simulink model "simulink_nodes"  (R2021a)
settings: Solver=VariableStepAuto  StartTime=0.0  StopTime=Episode_time  FixedStep=1e-4  MaxStep=TS  RelTol=1e-4
model workspace (MAT data in the model file):
  SL_ROS_VariableLengthArrays_MaxSizes.CommonInfo.ArrayTruncateAction = 'EmitWarning'
  SL_ROS_VariableLengthArrays_MaxSizes.MsgTypeMap = containers.Map
  SL_ROS_VariableLengthArrays_MaxSizes.MsgTypeMap.serialization.keys = {'std_msgs/Float32MultiArray', 'std_msgs/MultiArrayDimension'}
  SL_ROS_VariableLengthArrays_MaxSizes.MsgTypeMap.serialization.values{1}.PropertyName = 'Data'
  SL_ROS_VariableLengthArrays_MaxSizes.MsgTypeMap.serialization.values{1}.DataType = 'single'
  SL_ROS_VariableLengthArrays_MaxSizes.MsgTypeMap.serialization.values{1}.MaxLength = 4
  SL_ROS_VariableLengthArrays_MaxSizes.MsgTypeMap.serialization.values{2}.PropertyName = 'Label'
  SL_ROS_VariableLengthArrays_MaxSizes.MsgTypeMap.serialization.values{2}.DataType = 'uint8'
  SL_ROS_VariableLengthArrays_MaxSizes.MsgTypeMap.serialization.values{2}.MaxLength = 4
  SL_ROS_VariableLengthArrays_MaxSizes.MsgTypeMap.serialization.uniformity = 0
  SL_ROS_VariableLengthArrays_MaxSizes.MsgTypeMap.serialization.keyType = 'char'
  SL_ROS_VariableLengthArrays_MaxSizes.MsgTypeMap.serialization.valueType = 'any'
values from neighbouring files (symbols this model uses):
  Episode_time = 4    [matlab_node.m]
undefined symbols (not defined in the file or in its folder): Data, Data_SL_Info, X, Y, Z
libraries: sm_lib x10, robotlib x7, nesl_utility x6, simulink x1
settings Model: Creator=giulio  LastModifiedBy=giulio
settings SolverCC: NumberNewtonIterations=4  SolverResetMethod=Robust
settings OptimizationCC: EnhancedBackFolding=on  PassReuseOutputArgsAs=Individual arguments  ZeroExternalMemoryAtStartup=off  ZeroInternalMemoryAtStartup=off  MaxStackSize=64  OptimizeBlockOrder=speed  DifferentSizesBufferReuse=on  OptimizationCustomize=off  EfficientTunableParamExpr=on
settings DebuggingCC: ParameterTunabilityLossMsg=error
settings HardwareCC: ProdBitPerPointer=32  ProdBitPerSizeT=32  ProdBitPerPtrDiffT=32  ProdLargestAtomicFloat=None  ProdIntDivRoundTo=Undefined  ProdEndianess=Unspecified  ProdWordSize=32  ProdHWDeviceType=Generic->Unspecified (assume 32-bit Generic)  UseEmbeddedCoderFeatures=off
settings SFSimCC: MATLABDynamicMemAlloc=off
settings RTWCC: SystemTargetFile=ert.tlc  HardwareBoard=Robot Operating System (ROS)  TLCOptions="-aInlineSetEventsForThisBaseRateFcn=TLC_FALSE -aSuppressMultiTaskScheduler=TLC_FALSE  -aRateBasedStepFcn=0"  TemplateMakefile=ert_default_tmf  Toolchain=Catkin  TargetLang=C++
settings CodeAppCC: ForceParamTrailComments=on  IgnoreCustomStorageClasses=off  OperatorAnnotations=on  SimulinkDataObjDesc=on  SFDataObjDesc=on  InsertBlockDesc=on
settings ERTTargetCC: SupportNonInlinedSFcns=on  ERTCustomFileTemplate=rostime_codertarget_file_process.tlc

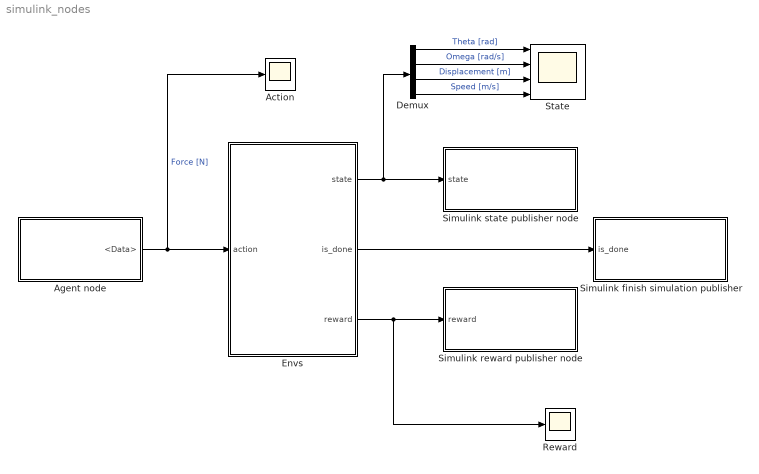
== system simulink_nodes ==
  Action : Scope
  Agent node : Subsystem
  Demux : Demux
  Envs : Subsystem
  Reward : Scope
  Simulink finish simulation publisher : Subsystem
  Simulink reward publisher node : Subsystem
  Simulink state publisher node : Subsystem
  State : Scope  NumInputPorts=4
  wires:
  Envs/1(state) -> Demux/1, Simulink state publisher node/1(state)
  Envs/2(is_done) -> Simulink finish simulation publisher/1(is_done)
  Envs/3(reward) -> Reward/1, Simulink reward publisher node/1(reward)
  Agent node/1(<Data>) -> Action/1, Envs/1(action)  "Force [N]"
  Demux/1 -> State/1  "Theta [rad]"
  Demux/2 -> State/2  "Omega [rad/s]"
  Demux/3 -> State/3  "Displacement [m]"
  Demux/4 -> State/4  "Speed [m/s]"

== system simulink_nodes/Agent node ==
  Bus Selector : BusSelector  OutputSignals=Data
  Subscribe : robotlib/Subscribe  topicSource=Specify your own  topic=/agent_action  messageType=std_msgs/Float32  SampleTime=-1  legacyBusStruct=off  messageQueueLength=1
  Terminator : Terminator
  <Data> : Outport
  wires:
  Bus Selector/1 -> <Data>/1  "<Data>"
  Subscribe/1 -> Terminator/1
  Subscribe/2 -> Bus Selector/1

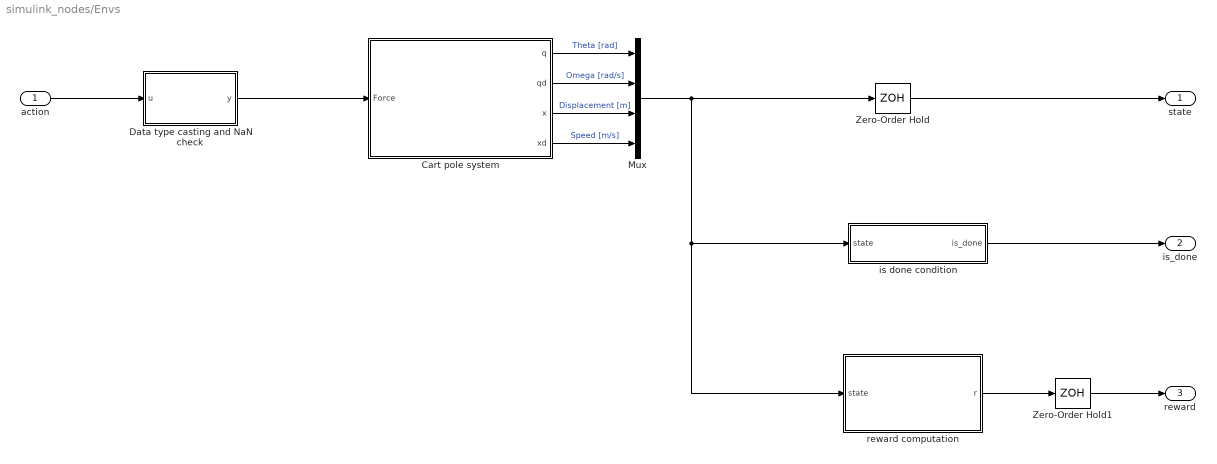
== system simulink_nodes/Envs ==
  action : Inport
  Cart pole system : Subsystem  mask(Cart pole system){mp=0.5, mc=3, bound=15, x_limit=0.5}
      mask prompts: mp "Pole mass [kg]"; mc "Cart pole [kg]"; bound "Pole boundaries [deg]"; x_limit "Cart boundaries [m]"
      mask help: Invertend pendulum on moving base.
      mask DialogControl ParameterGroupVar Prompt: System parameters
      mask Display: image('$imagefile'); % Use "Edit Image" on toolstrip to change.
  Data type casting and NaN check : Subsystem
  Mux : Mux
  Zero-Order Hold : ZeroOrderHold  SampleTime=-1
  Zero-Order Hold1 : ZeroOrderHold  SampleTime=-1
  is done condition : Subsystem  mask{T_sim=Episode_time, x_limit=0.5}
      mask prompts: T_sim "SImulation lenght [s]"; x_limit "X limit [m]"
  reward computation : Subsystem  mask{k_xdisp=100, k_error=20, x_limit=0.5, k_good_angle=10}
      mask prompts: k_xdisp "Displacement penality gain [-]"; k_error "Error angle penalty [-]"; x_limit "x limit [m]"; k_good_angle "Positive gain for good angle [-]"
  state : Outport
  is_done : Outport  Port=2
  reward : Outport  Port=3
  wires:
  Cart pole system/1(q) -> Mux/1  "Theta [rad]"
  Cart pole system/2(qd) -> Mux/2  "Omega [rad/s]"
  Cart pole system/3(x) -> Mux/3  "Displacement [m]"
  Cart pole system/4(xd) -> Mux/4  "Speed [m/s]"
  is done condition/1(is_done) -> is_done/1
  reward computation/1(r) -> Zero-Order Hold1/1
  Mux/1 -> reward computation/1(state), is done condition/1(state), Zero-Order Hold/1
  action/1 -> Data type casting and NaN check/1(u)
  Data type casting and NaN check/1(y) -> Cart pole system/1(Force)
  Zero-Order Hold/1 -> state/1
  Zero-Order Hold1/1 -> reward/1

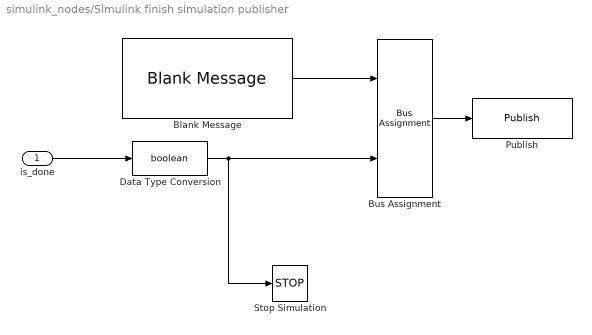
== system simulink_nodes/Simulink finish simulation publisher ==
  is_done : Inport
  Blank Message : robotlib/Blank Message  messageClass=Message  entityType=std_msgs/Bool  messageType=std_msgs/Bool  SampleTime=inf  legacyBusStruct=off
  Bus Assignment : BusAssignment  AssignedSignals=Data
  Data Type Conversion : DataTypeConversion  OutDataTypeStr=boolean
  Publish : robotlib/Publish  topicSource=Specify your own  topic=/is_done  messageType=std_msgs/Bool  legacyBusStruct=off  messageQueueLength=1
  Stop Simulation : Stop
  wires:
  Bus Assignment/1 -> Publish/1
  Blank Message/1 -> Bus Assignment/1
  is_done/1 -> Data Type Conversion/1
  Data Type Conversion/1 -> Stop Simulation/1, Bus Assignment/2

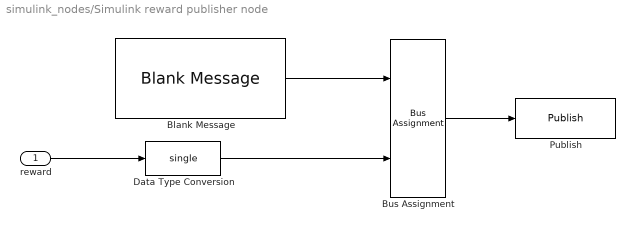
== system simulink_nodes/Simulink reward publisher node ==
  reward : Inport
  Blank Message : robotlib/Blank Message  messageClass=Message  entityType=std_msgs/Float32  messageType=std_msgs/Float32  SampleTime=inf  legacyBusStruct=off
  Bus Assignment : BusAssignment  AssignedSignals=Data
  Data Type Conversion : DataTypeConversion  OutDataTypeStr=single
  Publish : robotlib/Publish  topicSource=Specify your own  topic=/reward  messageType=std_msgs/Float32  legacyBusStruct=off  messageQueueLength=1
  wires:
  Data Type Conversion/1 -> Bus Assignment/2
  Blank Message/1 -> Bus Assignment/1
  Bus Assignment/1 -> Publish/1
  reward/1 -> Data Type Conversion/1

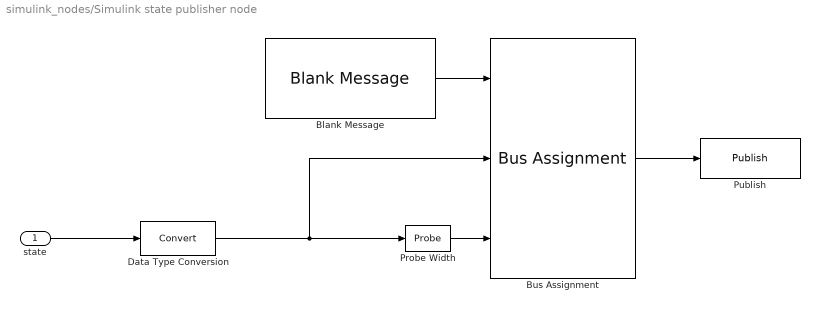
== system simulink_nodes/Simulink state publisher node ==
  state : Inport
  Blank Message : robotlib/Blank Message  messageClass=Message  entityType=std_msgs/Float32MultiArray  messageType=std_msgs/Float32MultiArray  SampleTime=inf  legacyBusStruct=off
  Bus Assignment : BusAssignment  AssignedSignals=Data,Data_SL_Info.CurrentLength
  Data Type Conversion : DataTypeConversion
  Probe Width : Probe  ProbeSampleTime=off  ProbeComplexSignal=off  ProbeWidthDataType=uint32
  Publish : robotlib/Publish  topicSource=Specify your own  topic=/state  messageType=std_msgs/Float32MultiArray  legacyBusStruct=off  messageQueueLength=1
  wires:
  Bus Assignment/1 -> Publish/1
  Probe Width/1 -> Bus Assignment/3
  Blank Message/1 -> Bus Assignment/1
  Data Type Conversion/1 -> Bus Assignment/2, Probe Width/1
  state/1 -> Data Type Conversion/1

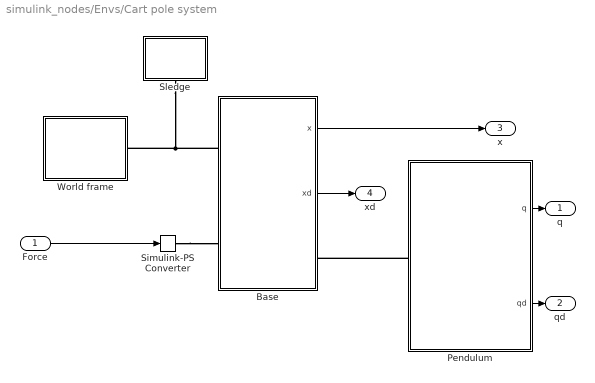
== system simulink_nodes/Envs/Cart pole system ==
  Force : Inport
  Base : Subsystem
  Pendulum : Subsystem
  Simulink-PS Converter : nesl_utility/Simulink-PS Converter  PhysicalDomain=network_engine_domain  SubClassName=ps_input  LeftPortType=input  RightPortType=output  PseudoPeriodic=off  Frequencies=[]  NoiseDistribution=none  NoiseParameters=[]  Unit=1  AffineConversion=off  FilteringAndDerivatives=filter  SimscapeFilterOrder=2  InputFilterTimeConstant=0.001  UdotUserProvided=0
      settings: SourceProductBaseCode=PW,SS
  Sledge : Subsystem
  World frame : Subsystem
  q : Outport
  qd : Outport  Port=2
  x : Outport  Port=3
  xd : Outport  Port=4
  wires:
  Pendulum/1(q) -> q/1
  Pendulum/2(qd) -> qd/1
  Base/2(xd) -> xd/1
  Force/1 -> Simulink-PS Converter/1
  Base/1(x) -> x/1
  connections:
  Simulink-PS Converter/RConn1 -- Base/LConn2
  Pendulum/LConn1 -- Base/RConn1
  Base/LConn1 -- World frame/RConn1 -- Sledge/LConn1

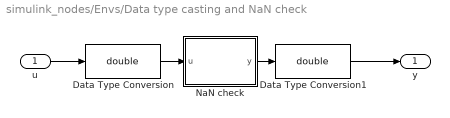
== system simulink_nodes/Envs/Data type casting and NaN check ==
  u : Inport
  Data Type Conversion : DataTypeConversion  OutDataTypeStr=double
  Data Type Conversion1 : DataTypeConversion  OutDataTypeStr=double
  NaN check : MATLAB Function  TreatAsAtomicUnit=on
  y : Outport
  wires:
  NaN check/1(y) -> Data Type Conversion1/1
  Data Type Conversion/1 -> NaN check/1(u)
  u/1 -> Data Type Conversion/1
  Data Type Conversion1/1 -> y/1

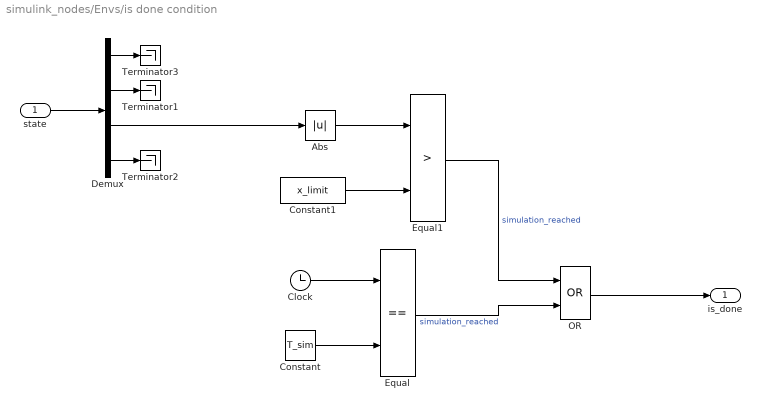
== system simulink_nodes/Envs/is done condition ==
  state : Inport
  Abs : Abs
  Clock : Clock
  Constant : Constant  Value=T_sim
  Constant1 : Constant  Value=x_limit
  Demux : Demux
  Equal : RelationalOperator  Operator===  OutDataTypeStr=boolean  RndMeth=Simplest
  Equal1 : RelationalOperator  Operator=>  OutDataTypeStr=boolean  RndMeth=Simplest
  OR : Logic  Operator=OR  AllPortsSameDT=off  OutDataTypeStr=boolean
  Terminator1 : Terminator
  Terminator2 : Terminator
  Terminator3 : Terminator
  is_done : Outport
  wires:
  Constant/1 -> Equal/2
  Clock/1 -> Equal/1
  state/1 -> Demux/1
  Equal/1 -> OR/2  "simulation_reached"
  OR/1 -> is_done/1
  Demux/3 -> Abs/1
  Abs/1 -> Equal1/1
  Constant1/1 -> Equal1/2
  Equal1/1 -> OR/1  "simulation_reached"
  Demux/2 -> Terminator1/1
  Demux/4 -> Terminator2/1
  Demux/1 -> Terminator3/1

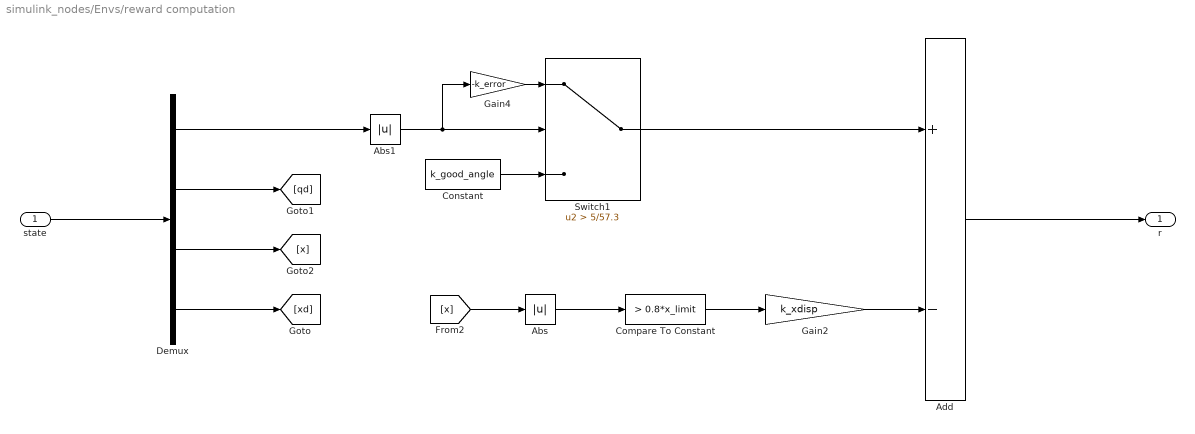
== system simulink_nodes/Envs/reward computation ==
  state : Inport
  Abs : Abs
  Abs1 : Abs
  Add : Sum  Inputs=+-
  Compare To Constant : simulink/Logic and Bit Operations/Compare To Constant  relop=>  const=0.8*x_limit  OutDataTypeStr=boolean
  Constant : Constant  Value=k_good_angle
  Demux : Demux
  Gain2 : Gain  Gain=k_xdisp
  Gain4 : Gain  Gain=-k_error
  Switch1 : Switch  Criteria=u2 > Threshold  Threshold=5/57.3
  r : Outport
  wires:
  state/1 -> Demux/1
  Abs/1 -> Compare To Constant/1
  Add/1 -> r/1
  Switch1/1 -> Add/1
  Demux/1 -> Abs1/1
  Demux/4 -> [xd]
  Demux/3 -> [x]
  Constant/1 -> Switch1/3
  Compare To Constant/1 -> Gain2/1
  Demux/2 -> [qd]
  [x] -> Abs/1
  Gain2/1 -> Add/2
  Abs1/1 -> Gain4/1, Switch1/2
  Gain4/1 -> Switch1/1

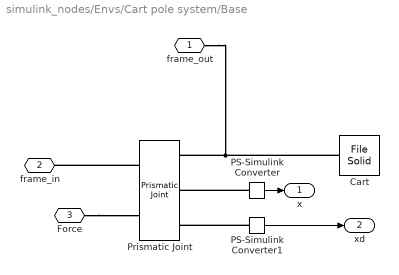
== system simulink_nodes/Envs/Cart pole system/Base ==
  Cart : sm_lib/Body Elements/File Solid  ExtGeomFileName=/home/giulio/rl_prj/simulink/BASE.STEP  UnitType=FromFile  ExtGeomFileUnits=m  StepReaderType=HEX  ExportConvexHullGeometry=off  InertiaType=PointMass  Mass=mc  MassUnits=kg  CenterOfMass=[0 0 0]  CenterOfMassUnits=m  MomentsOfInertia=[1 1 1]  MomentsOfInertiaUnits=kg*m^2  ProductsOfInertia=[0 0 0]  ProductsOfInertiaUnits=kg*m^2  BasedOnType=DensityFromFile  Density=1000  DensityUnits=kg/m^3  DoExposeReferenceFrame=on  SerializedFrames=<Frames/>  GraphicType=FromGeometry  MarkerShape=Sphere  MarkerSize=10  GraphicVisPropType=SimpleVisualProperties  GraphicDiffuseColor=[0.8 0.0 0.2]  GraphicSpecularColor=[0.5 0.5 0.5 1.0]  GraphicAmbientColor=[0.15 0.15 0.15 1.0]  GraphicEmissiveColor=[0.0 0.0 0.0 1.0]  GraphicShininess=75  GraphicOpacity=1.0
  PS-Simulink Converter : nesl_utility/PS-Simulink Converter  PhysicalDomain=network_engine_domain  SubClassName=ps_output  LeftPortType=input  RightPortType=output  PseudoPeriodic=off  Frequencies=[]  Unit=inherit  AffineConversion=off
      settings: SourceProductBaseCode=PW,SS
  PS-Simulink Converter1 : nesl_utility/PS-Simulink Converter  PhysicalDomain=network_engine_domain  SubClassName=ps_output  LeftPortType=input  RightPortType=output  PseudoPeriodic=off  Frequencies=[]  Unit=inherit  AffineConversion=off
      settings: SourceProductBaseCode=PW,SS
  Prismatic Joint : sm_lib/Joints/Prismatic Joint  JointMode=Normal  SenseConstraintForce=off  SenseConstraintForceX=off  SenseConstraintForceY=off  SenseConstraintForceZ=off  SenseConstraintTorque=off  SenseConstraintTorqueX=off  SenseConstraintTorqueY=off  SenseConstraintTorqueZ=off  SenseTotalForce=off  SenseTotalForceX=off  SenseTotalForceY=off  SenseTotalForceZ=off  SenseTotalTorque=off  SenseTotalTorqueX=off  SenseTotalTorqueY=off  SenseTotalTorqueZ=off  CompositeWrenchDir=FollowerOnBase  CompositeWrenchFrame=BaseFrame  EquilibriumPosition=0  EquilibriumPositionUnits=m  SpringStiffness=0  SpringStiffnessUnits=N/m  DampingCoefficient=0  DampingCoefficientUnits=N/(m/s)  TorqueActuationMode=InputTorque  MotionActuationMode=ComputedMotion  SensePosition=on  SenseVelocity=on  SenseAcceleration=off  SenseTorqueForce=off  SenseLowerLimitTorqueForce=off  SenseUpperLimitTorqueForce=off  LowerLimitSpecify=off  LowerLimitBound=-1  LowerLimitBoundUnits=m  LowerLimitStiffness=1e6  LowerLimitStiffnessUnits=N/m  LowerLimitDamping=1e3  LowerLimitDampingUnits=N/(m/s)  LowerLimitTransitionRegionWidth=1e-4  LowerLimitTransitionRegionWidthUnits=m  UpperLimitSpecify=off  UpperLimitBound=1  UpperLimitBoundUnits=m  UpperLimitStiffness=1e6  UpperLimitStiffnessUnits=N/m  UpperLimitDamping=1e3  UpperLimitDampingUnits=N/(m/s)  UpperLimitTransitionRegionWidth=1e-4  UpperLimitTransitionRegionWidthUnits=m  PositionTargetSpecify=on  PositionTargetPriority=Low  PositionTargetValue=0.4*x_limit*randn(1)  PositionTargetValueUnits=m  VelocityTargetSpecify=off  VelocityTargetPriority=Low  VelocityTargetValue=randn(1)  VelocityTargetValueUnits=m/s
  frame_out : PMIOPort  Side=Right
  frame_in : PMIOPort  Port=2  Side=Left
  Force : PMIOPort  Port=3  Side=Left
  x : Outport
  xd : Outport  Port=2
  wires:
  PS-Simulink Converter/1 -> x/1
  PS-Simulink Converter1/1 -> xd/1
  connections:
  Prismatic Joint/LConn1 -- frame_in/RConn1
  Force/RConn1 -- Prismatic Joint/LConn2
  frame_out/RConn1 -- Cart/RConn1 -- Prismatic Joint/RConn1
  PS-Simulink Converter/LConn1 -- Prismatic Joint/RConn2
  PS-Simulink Converter1/LConn1 -- Prismatic Joint/RConn3

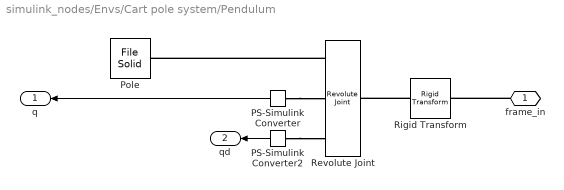
== system simulink_nodes/Envs/Cart pole system/Pendulum ==
  PS-Simulink Converter : nesl_utility/PS-Simulink Converter  PhysicalDomain=network_engine_domain  SubClassName=ps_output  LeftPortType=input  RightPortType=output  PseudoPeriodic=off  Frequencies=[]  Unit=inherit  AffineConversion=off
      settings: SourceProductBaseCode=PW,SS
  PS-Simulink Converter2 : nesl_utility/PS-Simulink Converter  PhysicalDomain=network_engine_domain  SubClassName=ps_output  LeftPortType=input  RightPortType=output  PseudoPeriodic=off  Frequencies=[]  Unit=inherit  AffineConversion=off
      settings: SourceProductBaseCode=PW,SS
  Pole : sm_lib/Body Elements/File Solid  ExtGeomFileName=/home/giulio/rl_prj/simulink/PEND.STEP  UnitType=FromFile  ExtGeomFileUnits=m  StepReaderType=HEX  ExportConvexHullGeometry=off  InertiaType=CalculateFromGeometry  Mass=mp  MassUnits=kg  CenterOfMass=[0 0 0]  CenterOfMassUnits=m  MomentsOfInertia=[1 1 1]  MomentsOfInertiaUnits=kg*m^2  ProductsOfInertia=[0 0 0]  ProductsOfInertiaUnits=kg*m^2  BasedOnType=Mass  Density=1000  DensityUnits=kg/m^3  DoExposeReferenceFrame=on  SerializedFrames=<Frames/>  GraphicType=FromGeometry  MarkerShape=Sphere  MarkerSize=10  GraphicVisPropType=SimpleVisualProperties  GraphicDiffuseColor=[0.0 0.2 0.6]  GraphicSpecularColor=[0.5 0.5 0.5 1.0]  GraphicAmbientColor=[0.15 0.15 0.15 1.0]  GraphicEmissiveColor=[0.0 0.0 0.0 1.0]  GraphicShininess=75  GraphicOpacity=1.0
  Revolute Joint : sm_lib/Joints/Revolute Joint  JointMode=Normal  SenseConstraintForce=off  SenseConstraintForceX=off  SenseConstraintForceY=off  SenseConstraintForceZ=off  SenseConstraintTorque=off  SenseConstraintTorqueX=off  SenseConstraintTorqueY=off  SenseConstraintTorqueZ=off  SenseTotalForce=off  SenseTotalForceX=off  SenseTotalForceY=off  SenseTotalForceZ=off  SenseTotalTorque=off  SenseTotalTorqueX=off  SenseTotalTorqueY=off  SenseTotalTorqueZ=off  CompositeWrenchDir=FollowerOnBase  CompositeWrenchFrame=BaseFrame  EquilibriumPosition=0  EquilibriumPositionUnits=deg  SpringStiffness=0  SpringStiffnessUnits=N*m/deg  DampingCoefficient=0  DampingCoefficientUnits=N*m/(deg/s)  TorqueActuationMode=NoTorque  MotionActuationMode=ComputedMotion  SensePosition=on  SenseVelocity=on  SenseAcceleration=off  SenseTorqueForce=off  SenseLowerLimitTorqueForce=off  SenseUpperLimitTorqueForce=off  LowerLimitSpecify=on  LowerLimitBound=-bound  LowerLimitBoundUnits=deg  LowerLimitStiffness=1e4  LowerLimitStiffnessUnits=N*m/deg  LowerLimitDamping=10  LowerLimitDampingUnits=N*m/(deg/s)  LowerLimitTransitionRegionWidth=0.1  LowerLimitTransitionRegionWidthUnits=deg  UpperLimitSpecify=on  UpperLimitBound=bound  UpperLimitBoundUnits=deg  UpperLimitStiffness=1e4  UpperLimitStiffnessUnits=N*m/deg  UpperLimitDamping=10  UpperLimitDampingUnits=N*m/(deg/s)  UpperLimitTransitionRegionWidth=0.1  UpperLimitTransitionRegionWidthUnits=deg  PositionTargetSpecify=on  PositionTargetPriority=Low  PositionTargetValue=bound*randn(1)  PositionTargetValueUnits=deg  VelocityTargetSpecify=off  VelocityTargetPriority=Low  VelocityTargetValue=randn(1)  VelocityTargetValueUnits=deg/s
  Rigid Transform : sm_lib/Frames and Transforms/Rigid Transform  TranslationMethod=None  TranslationStandardOffset=0  TranslationLengthUnit=m  TranslationStandardAxis=+Z  TranslationCartesianOffset=[0 0 0]  TranslationROffset=0  TranslationROffsetUnits=m  TranslationZOffset=0  TranslationZOffsetUnits=m  TranslationThetaOffset=0  TranslationThetaOffsetUnits=deg  RotationMethod=StandardAxis  RotationAngleUnits=deg  RotationStandardAxis=+Y  RotationAngle=90  RotationArbitraryAxis=[0 0 1]  FollAlignAxisA=+X  BaseAlignAxisA=+Y  FollAlignAxisB=+Y  BaseAlignAxisB=+Z  RotationSequenceAxes=FollowerAxes  RotationSequence=XYX  RotationSequenceAngles=[0 0 0]  RotationSequenceAnglesUnits=deg  RotationMatrix=[1 0 0; 0 1 0; 0 0 1]
  frame_in : PMIOPort  Side=Left
  q : Outport
  qd : Outport  Port=2
  wires:
  PS-Simulink Converter2/1 -> qd/1
  PS-Simulink Converter/1 -> q/1
  connections:
  Revolute Joint/RConn1 -- Pole/RConn1
  PS-Simulink Converter/LConn1 -- Revolute Joint/RConn2
  PS-Simulink Converter2/LConn1 -- Revolute Joint/RConn3
  frame_in/RConn1 -- Rigid Transform/LConn1
  Rigid Transform/RConn1 -- Revolute Joint/LConn1

== system simulink_nodes/Envs/Cart pole system/Sledge ==
  Brick Solid : sm_lib/Body Elements/Brick Solid  GraphicAmbientColor=[0.15 0.15 0.15 1.0]  BasedOnType=Density  BrickDimensions=[0.002 0.02 (1.9*x_limit)]  BrickDimensionUnits=m  CenterOfMass=[0 0 0]  CenterOfMassUnits=m  GraphicDiffuseColor=[0.0 0.0 0.0]  Density=1000  DensityUnits=kg/m^3  DoExposeReferenceFrame=on  GraphicEmissiveColor=[0.0 0.0 0.0 1.0]  ExportEntireGeometry=off  SerializedFrames=<Frames/>  MarkerShape=Sphere  MarkerSize=10  GraphicType=FromGeometry  InertiaType=CalculateFromGeometry  Mass=1  MassUnits=kg  MomentsOfInertia=[1 1 1]  MomentsOfInertiaUnits=kg*m^2  GraphicOpacity=1.0  ProductsOfInertia=[0 0 0]  ProductsOfInertiaUnits=kg*m^2  GraphicShininess=75  GraphicSpecularColor=[0.5 0.5 0.5 1.0]  GraphicVisPropType=SimpleVisualProperties
  Rigid Transform1 : sm_lib/Frames and Transforms/Rigid Transform  TranslationMethod=StandardAxis  TranslationStandardOffset=7  TranslationLengthUnit=mm  TranslationStandardAxis=+X  TranslationCartesianOffset=[0 0 25]  TranslationROffset=0  TranslationROffsetUnits=m  TranslationZOffset=0  TranslationZOffsetUnits=m  TranslationThetaOffset=0  TranslationThetaOffsetUnits=deg  RotationMethod=None  RotationAngleUnits=deg  RotationStandardAxis=+X  RotationAngle=90  RotationArbitraryAxis=[0 0 1]  FollAlignAxisA=+X  BaseAlignAxisA=+Y  FollAlignAxisB=+Y  BaseAlignAxisB=+Z  RotationSequenceAxes=FollowerAxes  RotationSequence=XYX  RotationSequenceAngles=[0 0 0]  RotationSequenceAnglesUnits=deg  RotationMatrix=[1 0 0; 0 1 0; 0 0 1]
  WF : PMIOPort  Side=Left
  connections:
  Brick Solid/RConn1 -- Rigid Transform1/RConn1
  Rigid Transform1/LConn1 -- WF/RConn1

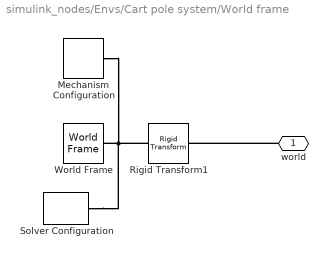
== system simulink_nodes/Envs/Cart pole system/World frame ==
  Mechanism Configuration : sm_lib/Utilities/Mechanism Configuration  UniformGravity=Constant  GravityVector=[0 0 -9.80665]  GravityVectorUnits=m/s^2  GravityUnits=m/s^2  LinearizationDelta=0.001  JointModeTransitionNonlinearIterations=2
  Rigid Transform1 : sm_lib/Frames and Transforms/Rigid Transform  TranslationMethod=None  TranslationStandardOffset=0  TranslationLengthUnit=mm  TranslationStandardAxis=+Z  TranslationCartesianOffset=[0 0 25]  TranslationROffset=0  TranslationROffsetUnits=m  TranslationZOffset=0  TranslationZOffsetUnits=m  TranslationThetaOffset=0  TranslationThetaOffsetUnits=deg  RotationMethod=StandardAxis  RotationAngleUnits=deg  RotationStandardAxis=+X  RotationAngle=90  RotationArbitraryAxis=[0 0 1]  FollAlignAxisA=+X  BaseAlignAxisA=+Y  FollAlignAxisB=+Y  BaseAlignAxisB=+Z  RotationSequenceAxes=FollowerAxes  RotationSequence=XYX  RotationSequenceAngles=[0 0 0]  RotationSequenceAnglesUnits=deg  RotationMatrix=[1 0 0; 0 1 0; 0 0 1]
  Solver Configuration : nesl_utility/Solver Configuration  PhysicalDomain=network_engine_domain  SubClassName=solver  LeftPortType=input  RightPortType=generic  Tones=[]  Harmonics=[]  SimulateNoise=off  Profile=off  UseLocalSampling=off  EnableSwitchedLinearOptims=on  FrequencyDomain=off  UseCCode=off  RelTol=0.001  AbsTol=1e-06  MinStep=1e-09  ToWorkspace=off  RevertToSquareIcSolve=off  NumHomotopyIterations=100  PhasorMode=off  PhasorModeNumHarmonics=1  DoDC=off  ResidualTolerance=1e-09  UseLocalSolver=off  LocalSolverChoice=NE_BACKWARD_EULER_ADVANCER  LocalSolverSampleTime=0.001  DoFixedCost=off  MaxNonlinIter=3  MaxModeIter=2  ComputeImpulses=off  ImpulseIterations=2  LinearAlgebra=auto  EquationFormulation=NE_TIME_EF  DelaysMemoryBudget=1024  AutomaticFiltering=on  FilteringTimeConstant=0.001  PartitionStorageMethod=AS_NEEDED  PartitionMemoryBudget=1024  PartitionMethod=ROBUST
      settings: SourceProductBaseCode=PW,SS
  World Frame : sm_lib/Frames and Transforms/World Frame
  world : PMIOPort  Side=Right
  connections:
  World Frame/RConn1 -- Rigid Transform1/LConn1 -- Solver Configuration/RConn1 -- Mechanism Configuration/RConn1
  world/RConn1 -- Rigid Transform1/RConn1

== matlab function simulink_nodes/Envs/Data type casting and NaN check/NaN check ==
  data: u input; y output
function y = fcn(u)

T = isnan(u);

if T == true
    y = 0;
    disp('is NaN. Output is ', y)
else
    y = u;
end
